simulink model "MatlabFunction_TestGen_cumsum3"  (R2017b)
settings: Solver=FixedStepDiscrete  StartTime=0.0  StopTime=10.0  RelTol=1e-3
settings Model: Creator=ktrinh  LastModifiedBy=ktrinh
settings DebuggingCC: ParameterOverflowMsg=none

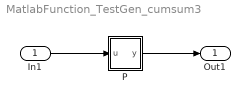
== system MatlabFunction_TestGen_cumsum3 ==
  In1 : Inport  OutDataTypeStr=int8  PortDimensions=[1,3]
  P : MATLAB Function  TreatAsAtomicUnit=on
  Out1 : Outport
  wires:
  In1/1 -> P/1(u)
  P/1(y) -> Out1/1

== matlab function MatlabFunction_TestGen_cumsum3/P ==
  data: u input; y output
function y = fcn(u)
y = cumsum(u);
